simulink model "MHILSimHWImpl"  (R2024a)
settings: Solver=FixedStepDiscrete  StartTime=0.0  StopTime=2e-4  FixedStep=4e-9  RelTol=1e-3
values from neighbouring files (symbols this model uses):
  cfg = tddbl_model    [HILSimModel.m]
undefined symbols (not defined in the file or in its folder): AXI4, dt, hw, ip, Lite, xc7z020clg400
libraries: hdlBasic x1497, hdlUtilities x3, vmcUtilities x1
(part 6 of 11)

== system MHILSimHWImpl/hilsim_ipcore/proc_domain/dac_nlf/nlf_dac1 ==
  note: Signal should now be normalized
      | to range -1 to 1.
  x : Inport
  presc : Inport  Port=2
  gain : Inport  Port=3
  cfg_select : Inport  Port=4
  cfg_addr : Inport  Port=5
  cfg_data : Inport  Port=6
  cfg_we : Inport  Port=7
  AddSub : hdlBasic/AddSub  mode=Addition  use_carryin=off  use_carryout=off  en=off  latency=1  precision=User Defined  arith_type=Unsigned  n_bits=ip.f_nlf.lut_addr_bits  bin_pt=0  quantization=Truncate  overflow=Wrap  use_behavioral_HDL=off  hw_selection=Fabric  pipelined=off  XmcBlockStatus=1  maskContainerNames=tabcontainer1  block_type=addsub  block_config=sysgen:Addsub_config
  AddSub1 : hdlBasic/AddSub  mode=Subtraction  use_carryin=off  use_carryout=off  en=off  latency=2  precision=User Defined  arith_type="Signed  (2's comp)"  n_bits=dt.slice.sz  bin_pt=dt.slice.bin  quantization=Truncate  overflow=Wrap  use_behavioral_HDL=off  hw_selection=Fabric  pipelined=off  XmcBlockStatus=1  maskContainerNames=tabcontainer1  block_type=addsub  block_config=sysgen:Addsub_config
  LUT : hdlBasic/Dual Port RAM  depth=ip.f_nlf.lut_sz  initVector=cfg.dac1_nlf.lut  distributed_mem=Block RAM  init_a=0  init_b=0  rst_a=off  rst_b=off  en_a=off  en_b=off  latency=1  write_mode_A=Read After Write  write_mode_B=Read After Write  explicit_period=[]  period=[]  simulation_type=fast_sim  XmcBlockStatus=1  maskContainerNames=tabcontainer1  block_type=dpram  block_config=sysgen:Dpram_config  optimize=Area
      settings: infoedit=[]
  Reinterpret : hdlBasic/Reinterpret  force_arith_type=on  arith_type=Unsigned  force_bin_pt=on  bin_pt=0  XmcBlockStatus=1  maskContainerNames=group1  block_type=reinterpret  block_config=sysgen:Reinterpret_config
  add_interpolate : hdlBasic/AddSub  mode=Addition  use_carryin=off  use_carryout=off  en=off  latency=1  precision=User Defined  arith_type="Signed  (2's comp)"  n_bits=dt.slice.sz  bin_pt=dt.slice.bin  quantization=Truncate  overflow=Wrap  use_behavioral_HDL=off  hw_selection=Fabric  pipelined=off  XmcBlockStatus=1  maskContainerNames=tabcontainer1  block_type=addsub  block_config=sysgen:Addsub_config
  addra_mux : hdlBasic/Mux  inputs=2  en=off  latency=1  precision=Full  arith_type=Unsigned  n_bits=16  bin_pt=14  quantization=Truncate  overflow=Wrap  XmcBlockStatus=1  maskContainerNames=tabcontainer1  block_type=mux  block_config=sysgen:Mux_config
  bool_zero_we : hdlBasic/Constant  const=0  gui_display_data_type=Boolean  arith_type=Boolean  n_bits=16  bin_pt=14  preci_type=Single  exp_width=8  frac_width=24  explicit_period=off  period=1  XmcBlockStatus=1  maskContainerNames=tabcontainer1  block_type=constant  block_config=sysgen:Constant_config
  bool_zero_wea : hdlBasic/Constant  const=0  gui_display_data_type=Boolean  arith_type=Boolean  n_bits=16  bin_pt=14  preci_type=Single  exp_width=8  frac_width=24  explicit_period=off  period=1  XmcBlockStatus=1  maskContainerNames=tabcontainer1  block_type=constant  block_config=sysgen:Constant_config
  cast_cutoff_lsbits : hdlBasic/Convert  gui_display_data_type=Fixed-point  arith_type=Signed (2's comp)  n_bits=ip.f_nlf.lut_addr_bits  bin_pt=ip.f_nlf.lut_addr_bits-1  float_type=Single  exp_bits=8  fraction_bits=24  quantization=Truncate  overflow=Wrap  en=off  latency=0  pipeline=off  XmcBlockStatus=1  maskContainerNames=group2  block_type=convert  block_config=sysgen:Convert_config  block_width=595  block_height=885
  cast_to_dt/slice : hdlBasic/Convert  gui_display_data_type=Fixed-point  arith_type=Signed (2's comp)  n_bits=dt.slice.sz  bin_pt=dt.slice.bin  float_type=Single  exp_bits=8  fraction_bits=24  quantization=Truncate  overflow=Wrap  en=off  latency=0  pipeline=off  XmcBlockStatus=1  maskContainerNames=group2  block_type=convert  block_config=sysgen:Convert_config  block_width=595  block_height=885
  const_1 : hdlBasic/Constant  const=1.0  gui_display_data_type=Fixed-point  arith_type=Unsigned  n_bits=ip.f_nlf.lut_addr_bits  bin_pt=0  preci_type=Single  exp_width=8  frac_width=24  explicit_period=off  period=1  XmcBlockStatus=1  maskContainerNames=tabcontainer1  block_type=constant  block_config=sysgen:Constant_config
  const_1_interp : hdlBasic/Constant  const=1  gui_display_data_type=Fixed-point  arith_type=Signed (2's comp)  n_bits=dt.slice.sz  bin_pt=dt.slice.bin  preci_type=Single  exp_width=8  frac_width=24  explicit_period=off  period=1  XmcBlockStatus=1  maskContainerNames=tabcontainer1  block_type=constant  block_config=sysgen:Constant_config
  cutoff_msbits : hdlBasic/Slice  nbits=dt.slice.bin - ip.f_nlf.lut_addr_bits + 1  boolean_output=off  mode=Lower Bit Location + Width  bit1=0  base1=MSB of Input  bit0=0  base0=LSB of Input  XmcBlockStatus=1  maskContainerNames=group1  block_type=slice  block_config=sysgen:Slice_config
  delay_sync_interpolate : hdlBasic/Delay  rst=off  en=off  latency=2  reg_retiming=off  XmcBlockStatus=1  maskContainerNames=group1  block_type=delay  block_config=sysgen:Delay_config
  dina_mux : hdlBasic/Mux  inputs=2  en=off  latency=1  precision=Full  arith_type=Unsigned  n_bits=16  bin_pt=14  quantization=Truncate  overflow=Wrap  XmcBlockStatus=1  maskContainerNames=tabcontainer1  block_type=mux  block_config=sysgen:Mux_config
  mult_a : hdlBasic/Mult  precision=User Defined  arith_type="Signed  (2's comp)"  n_bits=dt.slice.sz  bin_pt=dt.slice.bin  quantization=Truncate  overflow=Wrap  en=off  latency=3  use_behavioral_HDL=off  opt=Speed  use_embedded=on  optimum_pipeline=off  pipeline=on  use_rpm=on  placement_style=Triangular  XmcBlockStatus=1  maskContainerNames=group1  block_type=mult  block_config=sysgen:Mult_config  block_width=598  block_height=876
  mult_b : hdlBasic/Mult  precision=User Defined  arith_type="Signed  (2's comp)"  n_bits=dt.slice.sz  bin_pt=dt.slice.bin  quantization=Truncate  overflow=Wrap  en=off  latency=3  use_behavioral_HDL=off  opt=Speed  use_embedded=on  optimum_pipeline=off  pipeline=on  use_rpm=on  placement_style=Triangular  XmcBlockStatus=1  maskContainerNames=group1  block_type=mult  block_config=sysgen:Mult_config  block_width=598  block_height=876
  mult_inp_scale : hdlBasic/Mult  precision=User Defined  arith_type="Signed  (2's comp)"  n_bits=dt.slice.sz  bin_pt=dt.slice.sz - 2  quantization=Truncate  overflow=Wrap  en=off  latency=3  use_behavioral_HDL=off  opt=Speed  use_embedded=on  optimum_pipeline=off  pipeline=on  use_rpm=on  placement_style=Triangular  XmcBlockStatus=1  maskContainerNames=group1  block_type=mult  block_config=sysgen:Mult_config  block_width=598  block_height=876
  mult_out_scale : hdlBasic/Mult  precision=User Defined  arith_type="Signed  (2's comp)"  n_bits=dt.slice.sz  bin_pt=dt.slice.bin  quantization=Truncate  overflow=Wrap  en=off  latency=3  use_behavioral_HDL=off  opt=Speed  use_embedded=on  optimum_pipeline=off  pipeline=on  use_rpm=on  placement_style=Triangular  XmcBlockStatus=1  maskContainerNames=group1  block_type=mult  block_config=sysgen:Mult_config  block_width=598  block_height=876
  reint_sliced : hdlBasic/Reinterpret  force_arith_type=on  arith_type=Unsigned  force_bin_pt=on  bin_pt=dt.slice.bin - ip.f_nlf.lut_addr_bits + 1  XmcBlockStatus=1  maskContainerNames=group1  block_type=reinterpret  block_config=sysgen:Reinterpret_config
  wea_mux : hdlBasic/Mux  inputs=2  en=off  latency=1  precision=Full  arith_type=Unsigned  n_bits=16  bin_pt=14  quantization=Truncate  overflow=Wrap  XmcBlockStatus=1  maskContainerNames=tabcontainer1  block_type=mux  block_config=sysgen:Mux_config
  zero_nlf_datatype : hdlBasic/Constant  const=0  gui_display_data_type=Fixed-point  arith_type=Signed (2's comp)  n_bits=dt.nlf.sz  bin_pt=dt.nlf.bin  preci_type=Single  exp_width=8  frac_width=24  explicit_period=off  period=1  XmcBlockStatus=1  maskContainerNames=tabcontainer1  block_type=constant  block_config=sysgen:Constant_config
  zero_nlf_dina : hdlBasic/Constant  const=0  gui_display_data_type=Fixed-point  arith_type=Signed (2's comp)  n_bits=dt.nlf.sz  bin_pt=dt.nlf.bin  preci_type=Single  exp_width=8  frac_width=24  explicit_period=off  period=1  XmcBlockStatus=1  maskContainerNames=tabcontainer1  block_type=constant  block_config=sysgen:Constant_config
  f(x) : Outport
  wires:
  x/1 -> mult_inp_scale/1
  presc/1 -> mult_inp_scale/2
  cast_cutoff_lsbits/1 -> Reinterpret/1
  Reinterpret/1 -> addra_mux/2, AddSub/1
  const_1/1 -> AddSub/2
  AddSub/1 -> LUT/4
  bool_zero_we/1 -> LUT/6
  zero_nlf_datatype/1 -> LUT/5
  LUT/2 -> mult_b/1
  LUT/1 -> mult_a/1
  mult_inp_scale/1 -> cast_cutoff_lsbits/1, cutoff_msbits/1
  cutoff_msbits/1 -> reint_sliced/1
  reint_sliced/1 -> cast_to_dt/slice/1
  cast_to_dt/slice/1 -> AddSub1/2, delay_sync_interpolate/1
  const_1_interp/1 -> AddSub1/1
  delay_sync_interpolate/1 -> mult_b/2
  AddSub1/1 -> mult_a/2
  mult_a/1 -> add_interpolate/1
  mult_b/1 -> add_interpolate/2
  gain/1 -> mult_out_scale/2
  add_interpolate/1 -> mult_out_scale/1
  mult_out_scale/1 -> f(x)/1
  dina_mux/1 -> LUT/2
  addra_mux/1 -> LUT/1
  wea_mux/1 -> LUT/3
  bool_zero_wea/1 -> wea_mux/2
  zero_nlf_dina/1 -> dina_mux/2
  cfg_select/1 -> wea_mux/1, dina_mux/1, addra_mux/1
  cfg_addr/1 -> addra_mux/3
  cfg_data/1 -> dina_mux/3
  cfg_we/1 -> wea_mux/3

== system MHILSimHWImpl/hilsim_ipcore/proc_domain/output_matrix/nlf_dac0_xx0 ==
  note: Signal should now be normalized
      | to range -1 to 1.
  x : Inport
  presc : Inport  Port=2
  gain : Inport  Port=3
  cfg_select : Inport  Port=4
  cfg_addr : Inport  Port=5
  cfg_data : Inport  Port=6
  cfg_we : Inport  Port=7
  AddSub : hdlBasic/AddSub  mode=Addition  use_carryin=off  use_carryout=off  en=off  latency=1  precision=User Defined  arith_type=Unsigned  n_bits=ip.f_nlf.lut_addr_bits  bin_pt=0  quantization=Truncate  overflow=Wrap  use_behavioral_HDL=off  hw_selection=Fabric  pipelined=off  XmcBlockStatus=1  maskContainerNames=tabcontainer1  block_type=addsub  block_config=sysgen:Addsub_config
  AddSub1 : hdlBasic/AddSub  mode=Subtraction  use_carryin=off  use_carryout=off  en=off  latency=2  precision=User Defined  arith_type="Signed  (2's comp)"  n_bits=dt.slice.sz  bin_pt=dt.slice.bin  quantization=Truncate  overflow=Wrap  use_behavioral_HDL=off  hw_selection=Fabric  pipelined=off  XmcBlockStatus=1  maskContainerNames=tabcontainer1  block_type=addsub  block_config=sysgen:Addsub_config
  LUT : hdlBasic/Dual Port RAM  depth=ip.f_nlf.lut_sz  initVector=cfg.out_mat.nlf_dac0_xx0.lut  distributed_mem=Block RAM  init_a=0  init_b=0  rst_a=off  rst_b=off  en_a=off  en_b=off  latency=1  write_mode_A=Read After Write  write_mode_B=Read After Write  explicit_period=[]  period=[]  simulation_type=fast_sim  XmcBlockStatus=1  maskContainerNames=tabcontainer1  block_type=dpram  block_config=sysgen:Dpram_config  optimize=Area
      settings: infoedit=[]
  Reinterpret : hdlBasic/Reinterpret  force_arith_type=on  arith_type=Unsigned  force_bin_pt=on  bin_pt=0  XmcBlockStatus=1  maskContainerNames=group1  block_type=reinterpret  block_config=sysgen:Reinterpret_config
  add_interpolate : hdlBasic/AddSub  mode=Addition  use_carryin=off  use_carryout=off  en=off  latency=1  precision=User Defined  arith_type="Signed  (2's comp)"  n_bits=dt.slice.sz  bin_pt=dt.slice.bin  quantization=Truncate  overflow=Wrap  use_behavioral_HDL=off  hw_selection=Fabric  pipelined=off  XmcBlockStatus=1  maskContainerNames=tabcontainer1  block_type=addsub  block_config=sysgen:Addsub_config
  addra_mux : hdlBasic/Mux  inputs=2  en=off  latency=1  precision=Full  arith_type=Unsigned  n_bits=16  bin_pt=14  quantization=Truncate  overflow=Wrap  XmcBlockStatus=1  maskContainerNames=tabcontainer1  block_type=mux  block_config=sysgen:Mux_config
  bool_zero_we : hdlBasic/Constant  const=0  gui_display_data_type=Boolean  arith_type=Boolean  n_bits=16  bin_pt=14  preci_type=Single  exp_width=8  frac_width=24  explicit_period=off  period=1  XmcBlockStatus=1  maskContainerNames=tabcontainer1  block_type=constant  block_config=sysgen:Constant_config
  bool_zero_wea : hdlBasic/Constant  const=0  gui_display_data_type=Boolean  arith_type=Boolean  n_bits=16  bin_pt=14  preci_type=Single  exp_width=8  frac_width=24  explicit_period=off  period=1  XmcBlockStatus=1  maskContainerNames=tabcontainer1  block_type=constant  block_config=sysgen:Constant_config
  cast_cutoff_lsbits : hdlBasic/Convert  gui_display_data_type=Fixed-point  arith_type="Signed  (2's comp)"  n_bits=ip.f_nlf.lut_addr_bits  bin_pt=ip.f_nlf.lut_addr_bits-1  float_type=Single  exp_bits=8  fraction_bits=24  quantization=Truncate  overflow=Wrap  en=off  latency=0  pipeline=off  XmcBlockStatus=1  maskContainerNames=group2  block_type=convert  block_config=sysgen:Convert_config  block_width=595  block_height=885
  cast_to_dt/slice : hdlBasic/Convert  gui_display_data_type=Fixed-point  arith_type="Signed  (2's comp)"  n_bits=dt.slice.sz  bin_pt=dt.slice.bin  float_type=Single  exp_bits=8  fraction_bits=24  quantization=Truncate  overflow=Wrap  en=off  latency=0  pipeline=off  XmcBlockStatus=1  maskContainerNames=group2  block_type=convert  block_config=sysgen:Convert_config  block_width=595  block_height=885
  const_1 : hdlBasic/Constant  const=1.0  gui_display_data_type=Fixed-point  arith_type=Unsigned  n_bits=ip.f_nlf.lut_addr_bits  bin_pt=0  preci_type=Single  exp_width=8  frac_width=24  explicit_period=off  period=1  XmcBlockStatus=1  maskContainerNames=tabcontainer1  block_type=constant  block_config=sysgen:Constant_config
  const_1_interp : hdlBasic/Constant  const=1  gui_display_data_type=Fixed-point  arith_type=Signed (2's comp)  n_bits=dt.slice.sz  bin_pt=dt.slice.bin  preci_type=Single  exp_width=8  frac_width=24  explicit_period=off  period=1  XmcBlockStatus=1  maskContainerNames=tabcontainer1  block_type=constant  block_config=sysgen:Constant_config
  cutoff_msbits : hdlBasic/Slice  nbits=dt.slice.sz - ip.f_nlf.lut_addr_bits-1  boolean_output=off  mode=Lower Bit Location + Width  bit1=0  base1=MSB of Input  bit0=0  base0=LSB of Input  XmcBlockStatus=1  maskContainerNames=group1  block_type=slice  block_config=sysgen:Slice_config
  delay_sync_interpolate : hdlBasic/Delay  rst=off  en=off  latency=2  reg_retiming=off  XmcBlockStatus=1  maskContainerNames=group1  block_type=delay  block_config=sysgen:Delay_config
  dina_mux : hdlBasic/Mux  inputs=2  en=off  latency=1  precision=Full  arith_type=Unsigned  n_bits=16  bin_pt=14  quantization=Truncate  overflow=Wrap  XmcBlockStatus=1  maskContainerNames=tabcontainer1  block_type=mux  block_config=sysgen:Mux_config
  mult_a : hdlBasic/Mult  precision=User Defined  arith_type="Signed  (2's comp)"  n_bits=dt.slice.sz  bin_pt=dt.slice.bin  quantization=Truncate  overflow=Wrap  en=off  latency=3  opt_float=off  fp_mult_usage=No Usage  use_behavioral_HDL=off  opt=Speed  use_embedded=on  optimum_pipeline=off  pipeline=on  use_rpm=on  placement_style=Triangular  XmcBlockStatus=1  maskContainerNames=group1  block_type=mult  block_config=sysgen:Mult_config  block_width=598  block_height=876
  mult_b : hdlBasic/Mult  precision=User Defined  arith_type="Signed  (2's comp)"  n_bits=dt.slice.sz  bin_pt=dt.slice.bin  quantization=Truncate  overflow=Wrap  en=off  latency=3  opt_float=off  fp_mult_usage=No Usage  use_behavioral_HDL=off  opt=Speed  use_embedded=on  optimum_pipeline=off  pipeline=on  use_rpm=on  placement_style=Triangular  XmcBlockStatus=1  maskContainerNames=group1  block_type=mult  block_config=sysgen:Mult_config  block_width=598  block_height=876
  mult_inp_scale : hdlBasic/Mult  precision=User Defined  arith_type="Signed  (2's comp)"  n_bits=dt.slice.sz  bin_pt=dt.slice.sz - 2  quantization=Truncate  overflow=Wrap  en=off  latency=3  opt_float=off  fp_mult_usage=No Usage  use_behavioral_HDL=off  opt=Speed  use_embedded=on  optimum_pipeline=off  pipeline=on  use_rpm=on  placement_style=Triangular  XmcBlockStatus=1  maskContainerNames=group1  block_type=mult  block_config=sysgen:Mult_config  block_width=598  block_height=876
  mult_out_scale : hdlBasic/Mult  precision=User Defined  arith_type="Signed  (2's comp)"  n_bits=dt.slice.sz  bin_pt=dt.slice.bin  quantization=Truncate  overflow=Wrap  en=off  latency=3  opt_float=off  fp_mult_usage=No Usage  use_behavioral_HDL=off  opt=Speed  use_embedded=on  optimum_pipeline=off  pipeline=on  use_rpm=on  placement_style=Triangular  XmcBlockStatus=1  maskContainerNames=group1  block_type=mult  block_config=sysgen:Mult_config  block_width=598  block_height=876
  reint_sliced : hdlBasic/Reinterpret  force_arith_type=on  arith_type=Unsigned  force_bin_pt=on  bin_pt=dt.slice.sz - ip.f_nlf.lut_addr_bits-1  XmcBlockStatus=1  maskContainerNames=group1  block_type=reinterpret  block_config=sysgen:Reinterpret_config
  wea_mux : hdlBasic/Mux  inputs=2  en=off  latency=1  precision=Full  arith_type=Unsigned  n_bits=16  bin_pt=14  quantization=Truncate  overflow=Wrap  XmcBlockStatus=1  maskContainerNames=tabcontainer1  block_type=mux  block_config=sysgen:Mux_config
  zero_nlf_datatype : hdlBasic/Constant  const=0  gui_display_data_type=Fixed-point  arith_type=Signed (2's comp)  n_bits=dt.nlf.sz  bin_pt=dt.nlf.bin  preci_type=Single  exp_width=8  frac_width=24  explicit_period=off  period=1  XmcBlockStatus=1  maskContainerNames=tabcontainer1  block_type=constant  block_config=sysgen:Constant_config
  zero_nlf_dina : hdlBasic/Constant  const=0  gui_display_data_type=Fixed-point  arith_type=Signed (2's comp)  n_bits=dt.nlf.sz  bin_pt=dt.nlf.bin  preci_type=Single  exp_width=8  frac_width=24  explicit_period=off  period=1  XmcBlockStatus=1  maskContainerNames=tabcontainer1  block_type=constant  block_config=sysgen:Constant_config
  f(x) : Outport
  wires:
  x/1 -> mult_inp_scale/1
  presc/1 -> mult_inp_scale/2
  cast_cutoff_lsbits/1 -> Reinterpret/1
  Reinterpret/1 -> addra_mux/2, AddSub/1
  const_1/1 -> AddSub/2
  AddSub/1 -> LUT/4
  bool_zero_we/1 -> LUT/6
  zero_nlf_datatype/1 -> LUT/5
  LUT/2 -> mult_b/1
  LUT/1 -> mult_a/1
  mult_inp_scale/1 -> cast_cutoff_lsbits/1, cutoff_msbits/1
  cutoff_msbits/1 -> reint_sliced/1
  reint_sliced/1 -> cast_to_dt/slice/1
  cast_to_dt/slice/1 -> AddSub1/2, delay_sync_interpolate/1
  const_1_interp/1 -> AddSub1/1
  delay_sync_interpolate/1 -> mult_b/2
  AddSub1/1 -> mult_a/2
  mult_a/1 -> add_interpolate/1
  mult_b/1 -> add_interpolate/2
  gain/1 -> mult_out_scale/2
  mult_out_scale/1 -> f(x)/1
  dina_mux/1 -> LUT/2
  addra_mux/1 -> LUT/1
  wea_mux/1 -> LUT/3
  bool_zero_wea/1 -> wea_mux/2
  zero_nlf_dina/1 -> dina_mux/2
  cfg_select/1 -> wea_mux/1, dina_mux/1, addra_mux/1
  cfg_addr/1 -> addra_mux/3
  cfg_data/1 -> dina_mux/3
  cfg_we/1 -> wea_mux/3
  add_interpolate/1 -> mult_out_scale/1

== system MHILSimHWImpl/hilsim_ipcore/proc_domain/output_matrix/nlf_dac0_xx1 ==
  note: Signal should now be normalized
      | to range -1 to 1.
  x : Inport
  presc : Inport  Port=2
  gain : Inport  Port=3
  cfg_select : Inport  Port=4
  cfg_addr : Inport  Port=5
  cfg_data : Inport  Port=6
  cfg_we : Inport  Port=7
  AddSub : hdlBasic/AddSub  mode=Addition  use_carryin=off  use_carryout=off  en=off  latency=1  precision=User Defined  arith_type=Unsigned  n_bits=ip.f_nlf.lut_addr_bits  bin_pt=0  quantization=Truncate  overflow=Wrap  use_behavioral_HDL=off  hw_selection=Fabric  pipelined=off  XmcBlockStatus=1  maskContainerNames=tabcontainer1  block_type=addsub  block_config=sysgen:Addsub_config
  AddSub1 : hdlBasic/AddSub  mode=Subtraction  use_carryin=off  use_carryout=off  en=off  latency=2  precision=User Defined  arith_type="Signed  (2's comp)"  n_bits=dt.slice.sz  bin_pt=dt.slice.bin  quantization=Truncate  overflow=Wrap  use_behavioral_HDL=off  hw_selection=Fabric  pipelined=off  XmcBlockStatus=1  maskContainerNames=tabcontainer1  block_type=addsub  block_config=sysgen:Addsub_config
  LUT : hdlBasic/Dual Port RAM  depth=ip.f_nlf.lut_sz  initVector=cfg.out_mat.nlf_dac0_xx1.lut  distributed_mem=Block RAM  init_a=0  init_b=0  rst_a=off  rst_b=off  en_a=off  en_b=off  latency=1  write_mode_A=Read After Write  write_mode_B=Read After Write  explicit_period=[]  period=[]  simulation_type=fast_sim  XmcBlockStatus=1  maskContainerNames=tabcontainer1  block_type=dpram  block_config=sysgen:Dpram_config  optimize=Area
      settings: infoedit=[]
  Reinterpret : hdlBasic/Reinterpret  force_arith_type=on  arith_type=Unsigned  force_bin_pt=on  bin_pt=0  XmcBlockStatus=1  maskContainerNames=group1  block_type=reinterpret  block_config=sysgen:Reinterpret_config
  add_interpolate : hdlBasic/AddSub  mode=Addition  use_carryin=off  use_carryout=off  en=off  latency=1  precision=User Defined  arith_type="Signed  (2's comp)"  n_bits=dt.slice.sz  bin_pt=dt.slice.bin  quantization=Truncate  overflow=Wrap  use_behavioral_HDL=off  hw_selection=Fabric  pipelined=off  XmcBlockStatus=1  maskContainerNames=tabcontainer1  block_type=addsub  block_config=sysgen:Addsub_config
  addra_mux : hdlBasic/Mux  inputs=2  en=off  latency=1  precision=Full  arith_type=Unsigned  n_bits=16  bin_pt=14  quantization=Truncate  overflow=Wrap  XmcBlockStatus=1  maskContainerNames=tabcontainer1  block_type=mux  block_config=sysgen:Mux_config
  bool_zero_we : hdlBasic/Constant  const=0  gui_display_data_type=Boolean  arith_type=Boolean  n_bits=16  bin_pt=14  preci_type=Single  exp_width=8  frac_width=24  explicit_period=off  period=1  XmcBlockStatus=1  maskContainerNames=tabcontainer1  block_type=constant  block_config=sysgen:Constant_config
  bool_zero_wea : hdlBasic/Constant  const=0  gui_display_data_type=Boolean  arith_type=Boolean  n_bits=16  bin_pt=14  preci_type=Single  exp_width=8  frac_width=24  explicit_period=off  period=1  XmcBlockStatus=1  maskContainerNames=tabcontainer1  block_type=constant  block_config=sysgen:Constant_config
  cast_cutoff_lsbits : hdlBasic/Convert  gui_display_data_type=Fixed-point  arith_type="Signed  (2's comp)"  n_bits=ip.f_nlf.lut_addr_bits  bin_pt=ip.f_nlf.lut_addr_bits-1  float_type=Single  exp_bits=8  fraction_bits=24  quantization=Truncate  overflow=Wrap  en=off  latency=0  pipeline=off  XmcBlockStatus=1  maskContainerNames=group2  block_type=convert  block_config=sysgen:Convert_config  block_width=595  block_height=885
  cast_to_dt/slice : hdlBasic/Convert  gui_display_data_type=Fixed-point  arith_type="Signed  (2's comp)"  n_bits=dt.slice.sz  bin_pt=dt.slice.bin  float_type=Single  exp_bits=8  fraction_bits=24  quantization=Truncate  overflow=Wrap  en=off  latency=0  pipeline=off  XmcBlockStatus=1  maskContainerNames=group2  block_type=convert  block_config=sysgen:Convert_config  block_width=595  block_height=885
  const_1 : hdlBasic/Constant  const=1.0  gui_display_data_type=Fixed-point  arith_type=Unsigned  n_bits=ip.f_nlf.lut_addr_bits  bin_pt=0  preci_type=Single  exp_width=8  frac_width=24  explicit_period=off  period=1  XmcBlockStatus=1  maskContainerNames=tabcontainer1  block_type=constant  block_config=sysgen:Constant_config
  const_1_interp : hdlBasic/Constant  const=1  gui_display_data_type=Fixed-point  arith_type=Signed (2's comp)  n_bits=dt.slice.sz  bin_pt=dt.slice.bin  preci_type=Single  exp_width=8  frac_width=24  explicit_period=off  period=1  XmcBlockStatus=1  maskContainerNames=tabcontainer1  block_type=constant  block_config=sysgen:Constant_config
  cutoff_msbits : hdlBasic/Slice  nbits=dt.slice.sz - ip.f_nlf.lut_addr_bits-1  boolean_output=off  mode=Lower Bit Location + Width  bit1=0  base1=MSB of Input  bit0=0  base0=LSB of Input  XmcBlockStatus=1  maskContainerNames=group1  block_type=slice  block_config=sysgen:Slice_config
  delay_sync_interpolate : hdlBasic/Delay  rst=off  en=off  latency=2  reg_retiming=off  XmcBlockStatus=1  maskContainerNames=group1  block_type=delay  block_config=sysgen:Delay_config
  dina_mux : hdlBasic/Mux  inputs=2  en=off  latency=1  precision=Full  arith_type=Unsigned  n_bits=16  bin_pt=14  quantization=Truncate  overflow=Wrap  XmcBlockStatus=1  maskContainerNames=tabcontainer1  block_type=mux  block_config=sysgen:Mux_config
  mult_a : hdlBasic/Mult  precision=User Defined  arith_type="Signed  (2's comp)"  n_bits=dt.slice.sz  bin_pt=dt.slice.bin  quantization=Truncate  overflow=Wrap  en=off  latency=3  opt_float=off  fp_mult_usage=No Usage  use_behavioral_HDL=off  opt=Speed  use_embedded=on  optimum_pipeline=off  pipeline=on  use_rpm=on  placement_style=Triangular  XmcBlockStatus=1  maskContainerNames=group1  block_type=mult  block_config=sysgen:Mult_config  block_width=598  block_height=876
  mult_b : hdlBasic/Mult  precision=User Defined  arith_type="Signed  (2's comp)"  n_bits=dt.slice.sz  bin_pt=dt.slice.bin  quantization=Truncate  overflow=Wrap  en=off  latency=3  opt_float=off  fp_mult_usage=No Usage  use_behavioral_HDL=off  opt=Speed  use_embedded=on  optimum_pipeline=off  pipeline=on  use_rpm=on  placement_style=Triangular  XmcBlockStatus=1  maskContainerNames=group1  block_type=mult  block_config=sysgen:Mult_config  block_width=598  block_height=876
  mult_inp_scale : hdlBasic/Mult  precision=User Defined  arith_type="Signed  (2's comp)"  n_bits=dt.slice.sz  bin_pt=dt.slice.sz - 2  quantization=Truncate  overflow=Wrap  en=off  latency=3  opt_float=off  fp_mult_usage=No Usage  use_behavioral_HDL=off  opt=Speed  use_embedded=on  optimum_pipeline=off  pipeline=on  use_rpm=on  placement_style=Triangular  XmcBlockStatus=1  maskContainerNames=group1  block_type=mult  block_config=sysgen:Mult_config  block_width=598  block_height=876
  mult_out_scale : hdlBasic/Mult  precision=User Defined  arith_type="Signed  (2's comp)"  n_bits=dt.slice.sz  bin_pt=dt.slice.bin  quantization=Truncate  overflow=Wrap  en=off  latency=3  opt_float=off  fp_mult_usage=No Usage  use_behavioral_HDL=off  opt=Speed  use_embedded=on  optimum_pipeline=off  pipeline=on  use_rpm=on  placement_style=Triangular  XmcBlockStatus=1  maskContainerNames=group1  block_type=mult  block_config=sysgen:Mult_config  block_width=598  block_height=876
  reint_sliced : hdlBasic/Reinterpret  force_arith_type=on  arith_type=Unsigned  force_bin_pt=on  bin_pt=dt.slice.sz - ip.f_nlf.lut_addr_bits-1  XmcBlockStatus=1  maskContainerNames=group1  block_type=reinterpret  block_config=sysgen:Reinterpret_config
  wea_mux : hdlBasic/Mux  inputs=2  en=off  latency=1  precision=Full  arith_type=Unsigned  n_bits=16  bin_pt=14  quantization=Truncate  overflow=Wrap  XmcBlockStatus=1  maskContainerNames=tabcontainer1  block_type=mux  block_config=sysgen:Mux_config
  zero_nlf_datatype : hdlBasic/Constant  const=0  gui_display_data_type=Fixed-point  arith_type=Signed (2's comp)  n_bits=dt.nlf.sz  bin_pt=dt.nlf.bin  preci_type=Single  exp_width=8  frac_width=24  explicit_period=off  period=1  XmcBlockStatus=1  maskContainerNames=tabcontainer1  block_type=constant  block_config=sysgen:Constant_config
  zero_nlf_dina : hdlBasic/Constant  const=0  gui_display_data_type=Fixed-point  arith_type=Signed (2's comp)  n_bits=dt.nlf.sz  bin_pt=dt.nlf.bin  preci_type=Single  exp_width=8  frac_width=24  explicit_period=off  period=1  XmcBlockStatus=1  maskContainerNames=tabcontainer1  block_type=constant  block_config=sysgen:Constant_config
  f(x) : Outport
  wires:
  x/1 -> mult_inp_scale/1
  presc/1 -> mult_inp_scale/2
  cast_cutoff_lsbits/1 -> Reinterpret/1
  Reinterpret/1 -> addra_mux/2, AddSub/1
  const_1/1 -> AddSub/2
  AddSub/1 -> LUT/4
  bool_zero_we/1 -> LUT/6
  zero_nlf_datatype/1 -> LUT/5
  LUT/2 -> mult_b/1
  LUT/1 -> mult_a/1
  mult_inp_scale/1 -> cast_cutoff_lsbits/1, cutoff_msbits/1
  cutoff_msbits/1 -> reint_sliced/1
  reint_sliced/1 -> cast_to_dt/slice/1
  cast_to_dt/slice/1 -> AddSub1/2, delay_sync_interpolate/1
  const_1_interp/1 -> AddSub1/1
  delay_sync_interpolate/1 -> mult_b/2
  AddSub1/1 -> mult_a/2
  mult_a/1 -> add_interpolate/1
  mult_b/1 -> add_interpolate/2
  gain/1 -> mult_out_scale/2
  mult_out_scale/1 -> f(x)/1
  dina_mux/1 -> LUT/2
  addra_mux/1 -> LUT/1
  wea_mux/1 -> LUT/3
  bool_zero_wea/1 -> wea_mux/2
  zero_nlf_dina/1 -> dina_mux/2
  cfg_select/1 -> wea_mux/1, dina_mux/1, addra_mux/1
  cfg_addr/1 -> addra_mux/3
  cfg_data/1 -> dina_mux/3
  cfg_we/1 -> wea_mux/3
  add_interpolate/1 -> mult_out_scale/1

== system MHILSimHWImpl/hilsim_ipcore/proc_domain/output_matrix/nlf_dac0_xx2 ==
  note: Signal should now be normalized
      | to range -1 to 1.
  x : Inport
  presc : Inport  Port=2
  gain : Inport  Port=3
  cfg_select : Inport  Port=4
  cfg_addr : Inport  Port=5
  cfg_data : Inport  Port=6
  cfg_we : Inport  Port=7
  AddSub : hdlBasic/AddSub  mode=Addition  use_carryin=off  use_carryout=off  en=off  latency=1  precision=User Defined  arith_type=Unsigned  n_bits=ip.f_nlf.lut_addr_bits  bin_pt=0  quantization=Truncate  overflow=Wrap  use_behavioral_HDL=off  hw_selection=Fabric  pipelined=off  XmcBlockStatus=1  maskContainerNames=tabcontainer1  block_type=addsub  block_config=sysgen:Addsub_config
  AddSub1 : hdlBasic/AddSub  mode=Subtraction  use_carryin=off  use_carryout=off  en=off  latency=2  precision=User Defined  arith_type="Signed  (2's comp)"  n_bits=dt.slice.sz  bin_pt=dt.slice.bin  quantization=Truncate  overflow=Wrap  use_behavioral_HDL=off  hw_selection=Fabric  pipelined=off  XmcBlockStatus=1  maskContainerNames=tabcontainer1  block_type=addsub  block_config=sysgen:Addsub_config
  LUT : hdlBasic/Dual Port RAM  depth=ip.f_nlf.lut_sz  initVector=cfg.out_mat.nlf_dac0_xx2.lut  distributed_mem=Block RAM  init_a=0  init_b=0  rst_a=off  rst_b=off  en_a=off  en_b=off  latency=1  write_mode_A=Read After Write  write_mode_B=Read After Write  explicit_period=[]  period=[]  simulation_type=fast_sim  XmcBlockStatus=1  maskContainerNames=tabcontainer1  block_type=dpram  block_config=sysgen:Dpram_config  optimize=Area
      settings: infoedit=[]
  Reinterpret : hdlBasic/Reinterpret  force_arith_type=on  arith_type=Unsigned  force_bin_pt=on  bin_pt=0  XmcBlockStatus=1  maskContainerNames=group1  block_type=reinterpret  block_config=sysgen:Reinterpret_config
  add_interpolate : hdlBasic/AddSub  mode=Addition  use_carryin=off  use_carryout=off  en=off  latency=1  precision=User Defined  arith_type="Signed  (2's comp)"  n_bits=dt.slice.sz  bin_pt=dt.slice.bin  quantization=Truncate  overflow=Wrap  use_behavioral_HDL=off  hw_selection=Fabric  pipelined=off  XmcBlockStatus=1  maskContainerNames=tabcontainer1  block_type=addsub  block_config=sysgen:Addsub_config
  addra_mux : hdlBasic/Mux  inputs=2  en=off  latency=1  precision=Full  arith_type=Unsigned  n_bits=16  bin_pt=14  quantization=Truncate  overflow=Wrap  XmcBlockStatus=1  maskContainerNames=tabcontainer1  block_type=mux  block_config=sysgen:Mux_config
  bool_zero_we : hdlBasic/Constant  const=0  gui_display_data_type=Boolean  arith_type=Boolean  n_bits=16  bin_pt=14  preci_type=Single  exp_width=8  frac_width=24  explicit_period=off  period=1  XmcBlockStatus=1  maskContainerNames=tabcontainer1  block_type=constant  block_config=sysgen:Constant_config
  bool_zero_wea : hdlBasic/Constant  const=0  gui_display_data_type=Boolean  arith_type=Boolean  n_bits=16  bin_pt=14  preci_type=Single  exp_width=8  frac_width=24  explicit_period=off  period=1  XmcBlockStatus=1  maskContainerNames=tabcontainer1  block_type=constant  block_config=sysgen:Constant_config
  cast_cutoff_lsbits : hdlBasic/Convert  gui_display_data_type=Fixed-point  arith_type="Signed  (2's comp)"  n_bits=ip.f_nlf.lut_addr_bits  bin_pt=ip.f_nlf.lut_addr_bits-1  float_type=Single  exp_bits=8  fraction_bits=24  quantization=Truncate  overflow=Wrap  en=off  latency=0  pipeline=off  XmcBlockStatus=1  maskContainerNames=group2  block_type=convert  block_config=sysgen:Convert_config  block_width=595  block_height=885
  cast_to_dt/slice : hdlBasic/Convert  gui_display_data_type=Fixed-point  arith_type="Signed  (2's comp)"  n_bits=dt.slice.sz  bin_pt=dt.slice.bin  float_type=Single  exp_bits=8  fraction_bits=24  quantization=Truncate  overflow=Wrap  en=off  latency=0  pipeline=off  XmcBlockStatus=1  maskContainerNames=group2  block_type=convert  block_config=sysgen:Convert_config  block_width=595  block_height=885
  const_1 : hdlBasic/Constant  const=1.0  gui_display_data_type=Fixed-point  arith_type=Unsigned  n_bits=ip.f_nlf.lut_addr_bits  bin_pt=0  preci_type=Single  exp_width=8  frac_width=24  explicit_period=off  period=1  XmcBlockStatus=1  maskContainerNames=tabcontainer1  block_type=constant  block_config=sysgen:Constant_config
  const_1_interp : hdlBasic/Constant  const=1  gui_display_data_type=Fixed-point  arith_type=Signed (2's comp)  n_bits=dt.slice.sz  bin_pt=dt.slice.bin  preci_type=Single  exp_width=8  frac_width=24  explicit_period=off  period=1  XmcBlockStatus=1  maskContainerNames=tabcontainer1  block_type=constant  block_config=sysgen:Constant_config
  cutoff_msbits : hdlBasic/Slice  nbits=dt.slice.sz - ip.f_nlf.lut_addr_bits-1  boolean_output=off  mode=Lower Bit Location + Width  bit1=0  base1=MSB of Input  bit0=0  base0=LSB of Input  XmcBlockStatus=1  maskContainerNames=group1  block_type=slice  block_config=sysgen:Slice_config
  delay_sync_interpolate : hdlBasic/Delay  rst=off  en=off  latency=2  reg_retiming=off  XmcBlockStatus=1  maskContainerNames=group1  block_type=delay  block_config=sysgen:Delay_config
  dina_mux : hdlBasic/Mux  inputs=2  en=off  latency=1  precision=Full  arith_type=Unsigned  n_bits=16  bin_pt=14  quantization=Truncate  overflow=Wrap  XmcBlockStatus=1  maskContainerNames=tabcontainer1  block_type=mux  block_config=sysgen:Mux_config
  mult_a : hdlBasic/Mult  precision=User Defined  arith_type="Signed  (2's comp)"  n_bits=dt.slice.sz  bin_pt=dt.slice.bin  quantization=Truncate  overflow=Wrap  en=off  latency=3  opt_float=off  fp_mult_usage=No Usage  use_behavioral_HDL=off  opt=Speed  use_embedded=on  optimum_pipeline=off  pipeline=on  use_rpm=on  placement_style=Triangular  XmcBlockStatus=1  maskContainerNames=group1  block_type=mult  block_config=sysgen:Mult_config  block_width=598  block_height=876
  mult_b : hdlBasic/Mult  precision=User Defined  arith_type="Signed  (2's comp)"  n_bits=dt.slice.sz  bin_pt=dt.slice.bin  quantization=Truncate  overflow=Wrap  en=off  latency=3  opt_float=off  fp_mult_usage=No Usage  use_behavioral_HDL=off  opt=Speed  use_embedded=on  optimum_pipeline=off  pipeline=on  use_rpm=on  placement_style=Triangular  XmcBlockStatus=1  maskContainerNames=group1  block_type=mult  block_config=sysgen:Mult_config  block_width=598  block_height=876
  mult_inp_scale : hdlBasic/Mult  precision=User Defined  arith_type="Signed  (2's comp)"  n_bits=dt.slice.sz  bin_pt=dt.slice.sz - 2  quantization=Truncate  overflow=Wrap  en=off  latency=3  opt_float=off  fp_mult_usage=No Usage  use_behavioral_HDL=off  opt=Speed  use_embedded=on  optimum_pipeline=off  pipeline=on  use_rpm=on  placement_style=Triangular  XmcBlockStatus=1  maskContainerNames=group1  block_type=mult  block_config=sysgen:Mult_config  block_width=598  block_height=876
  mult_out_scale : hdlBasic/Mult  precision=User Defined  arith_type="Signed  (2's comp)"  n_bits=dt.slice.sz  bin_pt=dt.slice.bin  quantization=Truncate  overflow=Wrap  en=off  latency=3  opt_float=off  fp_mult_usage=No Usage  use_behavioral_HDL=off  opt=Speed  use_embedded=on  optimum_pipeline=off  pipeline=on  use_rpm=on  placement_style=Triangular  XmcBlockStatus=1  maskContainerNames=group1  block_type=mult  block_config=sysgen:Mult_config  block_width=598  block_height=876
  reint_sliced : hdlBasic/Reinterpret  force_arith_type=on  arith_type=Unsigned  force_bin_pt=on  bin_pt=dt.slice.sz - ip.f_nlf.lut_addr_bits-1  XmcBlockStatus=1  maskContainerNames=group1  block_type=reinterpret  block_config=sysgen:Reinterpret_config
  wea_mux : hdlBasic/Mux  inputs=2  en=off  latency=1  precision=Full  arith_type=Unsigned  n_bits=16  bin_pt=14  quantization=Truncate  overflow=Wrap  XmcBlockStatus=1  maskContainerNames=tabcontainer1  block_type=mux  block_config=sysgen:Mux_config
  zero_nlf_datatype : hdlBasic/Constant  const=0  gui_display_data_type=Fixed-point  arith_type=Signed (2's comp)  n_bits=dt.nlf.sz  bin_pt=dt.nlf.bin  preci_type=Single  exp_width=8  frac_width=24  explicit_period=off  period=1  XmcBlockStatus=1  maskContainerNames=tabcontainer1  block_type=constant  block_config=sysgen:Constant_config
  zero_nlf_dina : hdlBasic/Constant  const=0  gui_display_data_type=Fixed-point  arith_type=Signed (2's comp)  n_bits=dt.nlf.sz  bin_pt=dt.nlf.bin  preci_type=Single  exp_width=8  frac_width=24  explicit_period=off  period=1  XmcBlockStatus=1  maskContainerNames=tabcontainer1  block_type=constant  block_config=sysgen:Constant_config
  f(x) : Outport
  wires:
  x/1 -> mult_inp_scale/1
  presc/1 -> mult_inp_scale/2
  cast_cutoff_lsbits/1 -> Reinterpret/1
  Reinterpret/1 -> addra_mux/2, AddSub/1
  const_1/1 -> AddSub/2
  AddSub/1 -> LUT/4
  bool_zero_we/1 -> LUT/6
  zero_nlf_datatype/1 -> LUT/5
  LUT/2 -> mult_b/1
  LUT/1 -> mult_a/1
  mult_inp_scale/1 -> cast_cutoff_lsbits/1, cutoff_msbits/1
  cutoff_msbits/1 -> reint_sliced/1
  reint_sliced/1 -> cast_to_dt/slice/1
  cast_to_dt/slice/1 -> AddSub1/2, delay_sync_interpolate/1
  const_1_interp/1 -> AddSub1/1
  delay_sync_interpolate/1 -> mult_b/2
  AddSub1/1 -> mult_a/2
  mult_a/1 -> add_interpolate/1
  mult_b/1 -> add_interpolate/2
  gain/1 -> mult_out_scale/2
  mult_out_scale/1 -> f(x)/1
  dina_mux/1 -> LUT/2
  addra_mux/1 -> LUT/1
  wea_mux/1 -> LUT/3
  bool_zero_wea/1 -> wea_mux/2
  zero_nlf_dina/1 -> dina_mux/2
  cfg_select/1 -> wea_mux/1, dina_mux/1, addra_mux/1
  cfg_addr/1 -> addra_mux/3
  cfg_data/1 -> dina_mux/3
  cfg_we/1 -> wea_mux/3
  add_interpolate/1 -> mult_out_scale/1

== system MHILSimHWImpl/hilsim_ipcore/proc_domain/output_matrix/nlf_dac1_xx0 ==
  note: Signal should now be normalized
      | to range -1 to 1.
  x : Inport
  presc : Inport  Port=2
  gain : Inport  Port=3
  cfg_select : Inport  Port=4
  cfg_addr : Inport  Port=5
  cfg_data : Inport  Port=6
  cfg_we : Inport  Port=7
  AddSub : hdlBasic/AddSub  mode=Addition  use_carryin=off  use_carryout=off  en=off  latency=1  precision=User Defined  arith_type=Unsigned  n_bits=ip.f_nlf.lut_addr_bits  bin_pt=0  quantization=Truncate  overflow=Wrap  use_behavioral_HDL=off  hw_selection=Fabric  pipelined=off  XmcBlockStatus=1  maskContainerNames=tabcontainer1  block_type=addsub  block_config=sysgen:Addsub_config
  AddSub1 : hdlBasic/AddSub  mode=Subtraction  use_carryin=off  use_carryout=off  en=off  latency=2  precision=User Defined  arith_type="Signed  (2's comp)"  n_bits=dt.slice.sz  bin_pt=dt.slice.bin  quantization=Truncate  overflow=Wrap  use_behavioral_HDL=off  hw_selection=Fabric  pipelined=off  XmcBlockStatus=1  maskContainerNames=tabcontainer1  block_type=addsub  block_config=sysgen:Addsub_config
  LUT : hdlBasic/Dual Port RAM  depth=ip.f_nlf.lut_sz  initVector=cfg.out_mat.nlf_dac1_xx0.lut  distributed_mem=Block RAM  init_a=0  init_b=0  rst_a=off  rst_b=off  en_a=off  en_b=off  latency=1  write_mode_A=Read After Write  write_mode_B=Read After Write  explicit_period=[]  period=[]  simulation_type=fast_sim  XmcBlockStatus=1  maskContainerNames=tabcontainer1  block_type=dpram  block_config=sysgen:Dpram_config  optimize=Area
      settings: infoedit=[]
  Reinterpret : hdlBasic/Reinterpret  force_arith_type=on  arith_type=Unsigned  force_bin_pt=on  bin_pt=0  XmcBlockStatus=1  maskContainerNames=group1  block_type=reinterpret  block_config=sysgen:Reinterpret_config
  add_interpolate : hdlBasic/AddSub  mode=Addition  use_carryin=off  use_carryout=off  en=off  latency=1  precision=User Defined  arith_type="Signed  (2's comp)"  n_bits=dt.slice.sz  bin_pt=dt.slice.bin  quantization=Truncate  overflow=Wrap  use_behavioral_HDL=off  hw_selection=Fabric  pipelined=off  XmcBlockStatus=1  maskContainerNames=tabcontainer1  block_type=addsub  block_config=sysgen:Addsub_config
  addra_mux : hdlBasic/Mux  inputs=2  en=off  latency=1  precision=Full  arith_type=Unsigned  n_bits=16  bin_pt=14  quantization=Truncate  overflow=Wrap  XmcBlockStatus=1  maskContainerNames=tabcontainer1  block_type=mux  block_config=sysgen:Mux_config
  bool_zero_we : hdlBasic/Constant  const=0  gui_display_data_type=Boolean  arith_type=Boolean  n_bits=16  bin_pt=14  preci_type=Single  exp_width=8  frac_width=24  explicit_period=off  period=1  XmcBlockStatus=1  maskContainerNames=tabcontainer1  block_type=constant  block_config=sysgen:Constant_config
  bool_zero_wea : hdlBasic/Constant  const=0  gui_display_data_type=Boolean  arith_type=Boolean  n_bits=16  bin_pt=14  preci_type=Single  exp_width=8  frac_width=24  explicit_period=off  period=1  XmcBlockStatus=1  maskContainerNames=tabcontainer1  block_type=constant  block_config=sysgen:Constant_config
  cast_cutoff_lsbits : hdlBasic/Convert  gui_display_data_type=Fixed-point  arith_type="Signed  (2's comp)"  n_bits=ip.f_nlf.lut_addr_bits  bin_pt=ip.f_nlf.lut_addr_bits-1  float_type=Single  exp_bits=8  fraction_bits=24  quantization=Truncate  overflow=Wrap  en=off  latency=0  pipeline=off  XmcBlockStatus=1  maskContainerNames=group2  block_type=convert  block_config=sysgen:Convert_config  block_width=595  block_height=885
  cast_to_dt/slice : hdlBasic/Convert  gui_display_data_type=Fixed-point  arith_type="Signed  (2's comp)"  n_bits=dt.slice.sz  bin_pt=dt.slice.bin  float_type=Single  exp_bits=8  fraction_bits=24  quantization=Truncate  overflow=Wrap  en=off  latency=0  pipeline=off  XmcBlockStatus=1  maskContainerNames=group2  block_type=convert  block_config=sysgen:Convert_config  block_width=595  block_height=885
  const_1 : hdlBasic/Constant  const=1.0  gui_display_data_type=Fixed-point  arith_type=Unsigned  n_bits=ip.f_nlf.lut_addr_bits  bin_pt=0  preci_type=Single  exp_width=8  frac_width=24  explicit_period=off  period=1  XmcBlockStatus=1  maskContainerNames=tabcontainer1  block_type=constant  block_config=sysgen:Constant_config
  const_1_interp : hdlBasic/Constant  const=1  gui_display_data_type=Fixed-point  arith_type=Signed (2's comp)  n_bits=dt.slice.sz  bin_pt=dt.slice.bin  preci_type=Single  exp_width=8  frac_width=24  explicit_period=off  period=1  XmcBlockStatus=1  maskContainerNames=tabcontainer1  block_type=constant  block_config=sysgen:Constant_config
  cutoff_msbits : hdlBasic/Slice  nbits=dt.slice.sz - ip.f_nlf.lut_addr_bits-1  boolean_output=off  mode=Lower Bit Location + Width  bit1=0  base1=MSB of Input  bit0=0  base0=LSB of Input  XmcBlockStatus=1  maskContainerNames=group1  block_type=slice  block_config=sysgen:Slice_config
  delay_sync_interpolate : hdlBasic/Delay  rst=off  en=off  latency=2  reg_retiming=off  XmcBlockStatus=1  maskContainerNames=group1  block_type=delay  block_config=sysgen:Delay_config
  dina_mux : hdlBasic/Mux  inputs=2  en=off  latency=1  precision=Full  arith_type=Unsigned  n_bits=16  bin_pt=14  quantization=Truncate  overflow=Wrap  XmcBlockStatus=1  maskContainerNames=tabcontainer1  block_type=mux  block_config=sysgen:Mux_config
  mult_a : hdlBasic/Mult  precision=User Defined  arith_type="Signed  (2's comp)"  n_bits=dt.slice.sz  bin_pt=dt.slice.bin  quantization=Truncate  overflow=Wrap  en=off  latency=3  opt_float=off  fp_mult_usage=No Usage  use_behavioral_HDL=off  opt=Speed  use_embedded=on  optimum_pipeline=off  pipeline=on  use_rpm=on  placement_style=Triangular  XmcBlockStatus=1  maskContainerNames=group1  block_type=mult  block_config=sysgen:Mult_config  block_width=598  block_height=876
  mult_b : hdlBasic/Mult  precision=User Defined  arith_type="Signed  (2's comp)"  n_bits=dt.slice.sz  bin_pt=dt.slice.bin  quantization=Truncate  overflow=Wrap  en=off  latency=3  opt_float=off  fp_mult_usage=No Usage  use_behavioral_HDL=off  opt=Speed  use_embedded=on  optimum_pipeline=off  pipeline=on  use_rpm=on  placement_style=Triangular  XmcBlockStatus=1  maskContainerNames=group1  block_type=mult  block_config=sysgen:Mult_config  block_width=598  block_height=876
  mult_inp_scale : hdlBasic/Mult  precision=User Defined  arith_type="Signed  (2's comp)"  n_bits=dt.slice.sz  bin_pt=dt.slice.sz - 2  quantization=Truncate  overflow=Wrap  en=off  latency=3  opt_float=off  fp_mult_usage=No Usage  use_behavioral_HDL=off  opt=Speed  use_embedded=on  optimum_pipeline=off  pipeline=on  use_rpm=on  placement_style=Triangular  XmcBlockStatus=1  maskContainerNames=group1  block_type=mult  block_config=sysgen:Mult_config  block_width=598  block_height=876
  mult_out_scale : hdlBasic/Mult  precision=User Defined  arith_type="Signed  (2's comp)"  n_bits=dt.slice.sz  bin_pt=dt.slice.bin  quantization=Truncate  overflow=Wrap  en=off  latency=3  opt_float=off  fp_mult_usage=No Usage  use_behavioral_HDL=off  opt=Speed  use_embedded=on  optimum_pipeline=off  pipeline=on  use_rpm=on  placement_style=Triangular  XmcBlockStatus=1  maskContainerNames=group1  block_type=mult  block_config=sysgen:Mult_config  block_width=598  block_height=876
  reint_sliced : hdlBasic/Reinterpret  force_arith_type=on  arith_type=Unsigned  force_bin_pt=on  bin_pt=dt.slice.sz - ip.f_nlf.lut_addr_bits-1  XmcBlockStatus=1  maskContainerNames=group1  block_type=reinterpret  block_config=sysgen:Reinterpret_config
  wea_mux : hdlBasic/Mux  inputs=2  en=off  latency=1  precision=Full  arith_type=Unsigned  n_bits=16  bin_pt=14  quantization=Truncate  overflow=Wrap  XmcBlockStatus=1  maskContainerNames=tabcontainer1  block_type=mux  block_config=sysgen:Mux_config
  zero_nlf_datatype : hdlBasic/Constant  const=0  gui_display_data_type=Fixed-point  arith_type=Signed (2's comp)  n_bits=dt.nlf.sz  bin_pt=dt.nlf.bin  preci_type=Single  exp_width=8  frac_width=24  explicit_period=off  period=1  XmcBlockStatus=1  maskContainerNames=tabcontainer1  block_type=constant  block_config=sysgen:Constant_config
  zero_nlf_dina : hdlBasic/Constant  const=0  gui_display_data_type=Fixed-point  arith_type=Signed (2's comp)  n_bits=dt.nlf.sz  bin_pt=dt.nlf.bin  preci_type=Single  exp_width=8  frac_width=24  explicit_period=off  period=1  XmcBlockStatus=1  maskContainerNames=tabcontainer1  block_type=constant  block_config=sysgen:Constant_config
  f(x) : Outport
  wires:
  x/1 -> mult_inp_scale/1
  presc/1 -> mult_inp_scale/2
  cast_cutoff_lsbits/1 -> Reinterpret/1
  Reinterpret/1 -> addra_mux/2, AddSub/1
  const_1/1 -> AddSub/2
  AddSub/1 -> LUT/4
  bool_zero_we/1 -> LUT/6
  zero_nlf_datatype/1 -> LUT/5
  LUT/2 -> mult_b/1
  LUT/1 -> mult_a/1
  mult_inp_scale/1 -> cast_cutoff_lsbits/1, cutoff_msbits/1
  cutoff_msbits/1 -> reint_sliced/1
  reint_sliced/1 -> cast_to_dt/slice/1
  cast_to_dt/slice/1 -> AddSub1/2, delay_sync_interpolate/1
  const_1_interp/1 -> AddSub1/1
  delay_sync_interpolate/1 -> mult_b/2
  AddSub1/1 -> mult_a/2
  mult_a/1 -> add_interpolate/1
  mult_b/1 -> add_interpolate/2
  gain/1 -> mult_out_scale/2
  mult_out_scale/1 -> f(x)/1
  dina_mux/1 -> LUT/2
  addra_mux/1 -> LUT/1
  wea_mux/1 -> LUT/3
  bool_zero_wea/1 -> wea_mux/2
  zero_nlf_dina/1 -> dina_mux/2
  cfg_select/1 -> wea_mux/1, dina_mux/1, addra_mux/1
  cfg_addr/1 -> addra_mux/3
  cfg_data/1 -> dina_mux/3
  cfg_we/1 -> wea_mux/3
  add_interpolate/1 -> mult_out_scale/1
